simulink model "Assignment4"  (R2014a)
settings: Solver=FixedStepDiscrete  StartTime=0.0  StopTime=10.0  FixedStep=1  RelTol=1e-3
libraries: hdlsllib x16, simulink x4
settings Model: Creator=ramirezlara.h  LastModifiedBy=ramirezlara.h

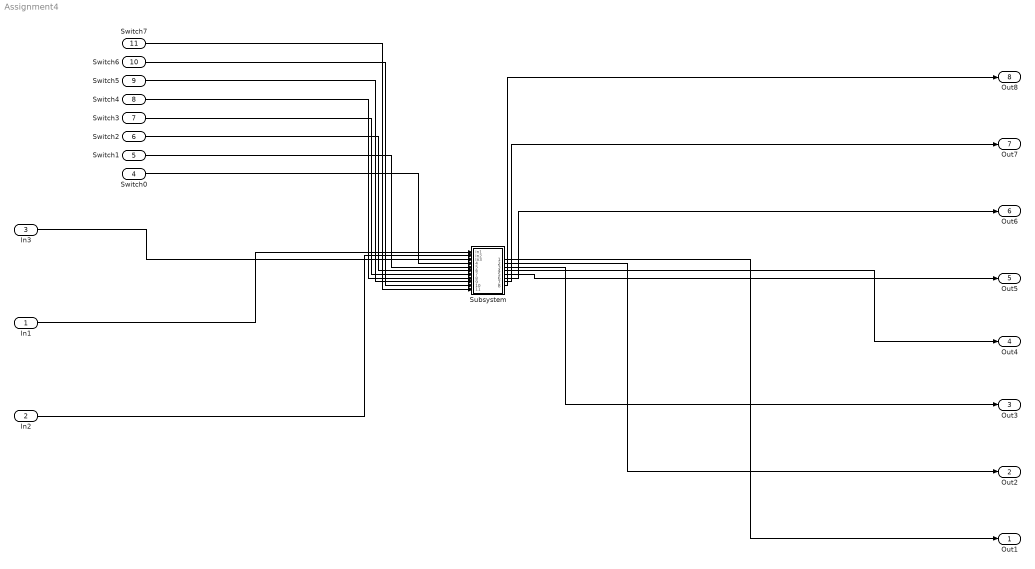
== system Assignment4 ==
  In1 : Inport
  In2 : Inport  Port=2
  In3 : Inport  Port=3
  Switch0 : Inport  Port=4
  Switch1 : Inport  Port=5
  Switch2 : Inport  Port=6
  Switch3 : Inport  Port=7
  Switch4 : Inport  Port=8
  Switch5 : Inport  Port=9
  Switch6 : Inport  Port=10
  Switch7 : Inport  Port=11
  Subsystem : Subsystem  TreatAsAtomicUnit=on
  Out1 : Outport
  Out2 : Outport  Port=2
  Out3 : Outport  Port=3
  Out4 : Outport  Port=4
  Out5 : Outport  Port=5
  Out6 : Outport  Port=6
  Out7 : Outport  Port=7
  Out8 : Outport  Port=8
  wires:
  In1/1 -> Subsystem/1(In1)
  In2/1 -> Subsystem/2(In2)
  In3/1 -> Subsystem/3(In3)
  Switch0/1 -> Subsystem/4(Switch0)
  Switch1/1 -> Subsystem/5(Switch1)
  Switch2/1 -> Subsystem/6(Switch2)
  Switch3/1 -> Subsystem/7(Switch3)
  Switch4/1 -> Subsystem/8(Switch4)
  Switch5/1 -> Subsystem/9(Switch5)
  Switch6/1 -> Subsystem/10(Switch6)
  Switch7/1 -> Subsystem/11(Switch7)
  Subsystem/1(Out1) -> Out1/1
  Subsystem/2(Out2) -> Out2/1
  Subsystem/3(Out3) -> Out3/1
  Subsystem/4(Out4) -> Out4/1
  Subsystem/5(Out5) -> Out5/1
  Subsystem/6(Out6) -> Out6/1
  Subsystem/7(Out7) -> Out7/1
  Subsystem/8(Out8) -> Out8/1

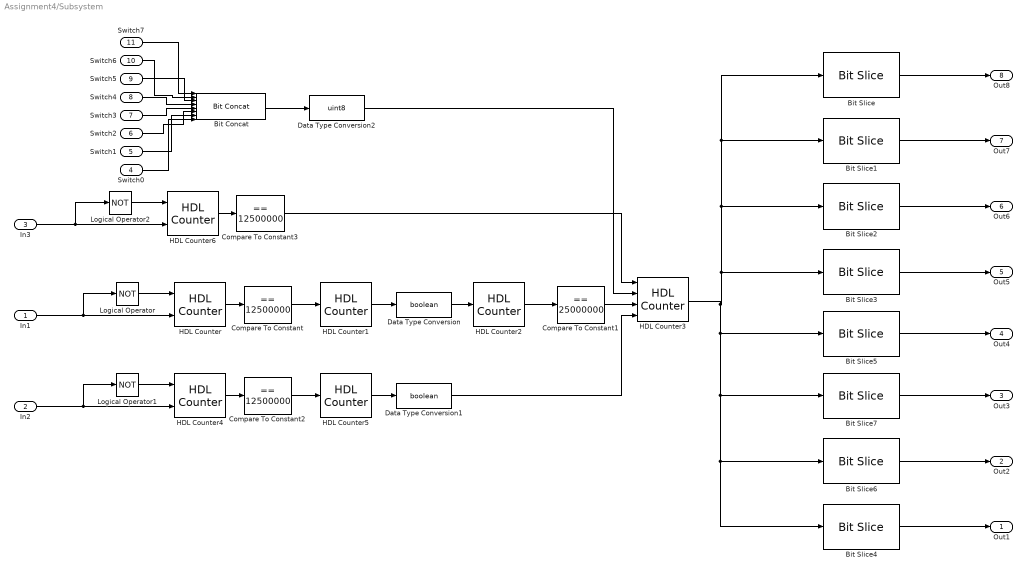
== system Assignment4/Subsystem ==
  In1 : Inport
  In2 : Inport  Port=2
  In3 : Inport  Port=3
  Switch0 : Inport  Port=4  OutDataTypeStr=boolean
  Switch1 : Inport  Port=5  OutDataTypeStr=boolean
  Switch2 : Inport  Port=6  OutDataTypeStr=boolean
  Switch3 : Inport  Port=7  OutDataTypeStr=boolean
  Switch4 : Inport  Port=8  OutDataTypeStr=boolean
  Switch5 : Inport  Port=9  OutDataTypeStr=boolean
  Switch6 : Inport  Port=10  OutDataTypeStr=boolean
  Switch7 : Inport  Port=11  OutDataTypeStr=boolean
  Bit Concat : hdlsllib/HDL Operations/Bit Concat  numInputs=8
  Bit Slice : hdlsllib/HDL Operations/Bit Slice  lidx=7  ridx=7
  Bit Slice1 : hdlsllib/HDL Operations/Bit Slice  lidx=6  ridx=6
  Bit Slice2 : hdlsllib/HDL Operations/Bit Slice  lidx=5  ridx=5
  Bit Slice3 : hdlsllib/HDL Operations/Bit Slice  lidx=4  ridx=4
  Bit Slice4 : hdlsllib/HDL Operations/Bit Slice  lidx=0  ridx=0
  Bit Slice5 : hdlsllib/HDL Operations/Bit Slice  lidx=3  ridx=3
  Bit Slice6 : hdlsllib/HDL Operations/Bit Slice  lidx=1  ridx=1
  Bit Slice7 : hdlsllib/HDL Operations/Bit Slice  lidx=2  ridx=2
  Compare To Constant : simulink/Logic and Bit Operations/Compare To Constant  relop===  const=12500000  OutDataTypeStr=boolean
  Compare To Constant1 : simulink/Logic and Bit Operations/Compare To Constant  relop===  const=25000000  OutDataTypeStr=boolean
  Compare To Constant2 : simulink/Logic and Bit Operations/Compare To Constant  relop===  const=12500000  OutDataTypeStr=boolean
  Compare To Constant3 : simulink/Logic and Bit Operations/Compare To Constant  relop===  const=12500000  OutDataTypeStr=boolean
  Data Type Conversion : DataTypeConversion  OutDataTypeStr=boolean
  Data Type Conversion1 : DataTypeConversion  OutDataTypeStr=boolean
  Data Type Conversion2 : DataTypeConversion  OutDataTypeStr=uint8
  HDL Counter : hdlsllib/HDL Operations/HDL Counter  CountType=Count limited  CountInit=0  CountStep=1  CountMax=50000000  CountFromType=Initial value  CountFrom=0  CountResetPort=on  CountLoadPort=off  CountEnbPort=on  CountDirPort=off  CountDataType=Unsigned  CountWordLen=32  CountFracLen=0  CountSampTime=1
  HDL Counter1 : hdlsllib/HDL Operations/HDL Counter  CountType=Free running  CountInit=0  CountStep=1  CountMax=100  CountFromType=Initial value  CountFrom=0  CountResetPort=off  CountLoadPort=off  CountEnbPort=on  CountDirPort=off  CountDataType=Unsigned  CountWordLen=1  CountFracLen=0  CountSampTime=1
  HDL Counter2 : hdlsllib/HDL Operations/HDL Counter  CountType=Count limited  CountInit=1  CountStep=1  CountMax=25000000  CountFromType=Initial value  CountFrom=1  CountResetPort=off  CountLoadPort=off  CountEnbPort=on  CountDirPort=off  CountDataType=Unsigned  CountWordLen=32  CountFracLen=0  CountSampTime=1
  HDL Counter3 : hdlsllib/HDL Operations/HDL Counter  CountType=Free running  CountInit=0  CountStep=1  CountMax=25000000  CountFromType=Initial value  CountFrom=0  CountResetPort=off  CountLoadPort=on  CountEnbPort=on  CountDirPort=on  CountDataType=Unsigned  CountWordLen=8  CountFracLen=0  CountSampTime=1
  HDL Counter4 : hdlsllib/HDL Operations/HDL Counter  CountType=Count limited  CountInit=0  CountStep=1  CountMax=50000000  CountFromType=Initial value  CountFrom=0  CountResetPort=on  CountLoadPort=off  CountEnbPort=on  CountDirPort=off  CountDataType=Unsigned  CountWordLen=32  CountFracLen=0  CountSampTime=1
  HDL Counter5 : hdlsllib/HDL Operations/HDL Counter  CountType=Free running  CountInit=1  CountStep=1  CountMax=100  CountFromType=Initial value  CountFrom=1  CountResetPort=off  CountLoadPort=off  CountEnbPort=on  CountDirPort=off  CountDataType=Unsigned  CountWordLen=1  CountFracLen=0  CountSampTime=1
  HDL Counter6 : hdlsllib/HDL Operations/HDL Counter  CountType=Count limited  CountInit=0  CountStep=1  CountMax=50000000  CountFromType=Initial value  CountFrom=0  CountResetPort=on  CountLoadPort=off  CountEnbPort=on  CountDirPort=off  CountDataType=Unsigned  CountWordLen=32  CountFracLen=0  CountSampTime=1
  Logical Operator : Logic  Operator=NOT  IconShape=distinctive  AllPortsSameDT=off  OutDataTypeStr=boolean
  Logical Operator1 : Logic  Operator=NOT  IconShape=distinctive  AllPortsSameDT=off  OutDataTypeStr=boolean
  Logical Operator2 : Logic  Operator=NOT  IconShape=distinctive  AllPortsSameDT=off  OutDataTypeStr=boolean
  Out1 : Outport
  Out2 : Outport  Port=2
  Out3 : Outport  Port=3
  Out4 : Outport  Port=4
  Out5 : Outport  Port=5
  Out6 : Outport  Port=6
  Out7 : Outport  Port=7
  Out8 : Outport  Port=8
  wires:
  HDL Counter4/1 -> Compare To Constant2/1
  Logical Operator1/1 -> HDL Counter4/1
  In2/1 -> HDL Counter4/2, Logical Operator1/1
  Compare To Constant2/1 -> HDL Counter5/1
  HDL Counter5/1 -> Data Type Conversion1/1
  Compare To Constant1/1 -> HDL Counter3/3
  Logical Operator/1 -> HDL Counter/1
  HDL Counter2/1 -> Compare To Constant1/1
  HDL Counter1/1 -> Data Type Conversion/1
  Data Type Conversion/1 -> HDL Counter2/1
  In1/1 -> HDL Counter/2, Logical Operator/1
  HDL Counter/1 -> Compare To Constant/1
  Compare To Constant/1 -> HDL Counter1/1
  HDL Counter3/1 -> Bit Slice2/1, Bit Slice1/1, Bit Slice/1, Bit Slice3/1, Bit Slice6/1, Bit Slice4/1, Bit Slice7/1, Bit Slice5/1
  Data Type Conversion1/1 -> HDL Counter3/4
  Compare To Constant3/1 -> HDL Counter3/1
  Bit Slice1/1 -> Out7/1
  Switch3/1 -> Bit Concat/5
  Bit Slice2/1 -> Out6/1
  Switch5/1 -> Bit Concat/3
  Logical Operator2/1 -> HDL Counter6/1
  Switch0/1 -> Bit Concat/8
  Bit Slice6/1 -> Out2/1
  Bit Slice3/1 -> Out5/1
  In3/1 -> HDL Counter6/2, Logical Operator2/1
  HDL Counter6/1 -> Compare To Constant3/1
  Switch2/1 -> Bit Concat/6
  Switch7/1 -> Bit Concat/1
  Switch4/1 -> Bit Concat/4
  Bit Slice5/1 -> Out4/1
  Switch6/1 -> Bit Concat/2
  Bit Slice/1 -> Out8/1
  Bit Slice7/1 -> Out3/1
  Bit Slice4/1 -> Out1/1
  Switch1/1 -> Bit Concat/7
  Bit Concat/1 -> Data Type Conversion2/1
  Data Type Conversion2/1 -> HDL Counter3/2
